simulink model "aves"  (R2012b)
settings: Solver=ode45  StartTime=0.0  StopTime=10.0  RelTol=1e-3
undefined symbols (not defined in the file): ave
settings Model: Creator=Daniel  LastModifiedBy=Daniel

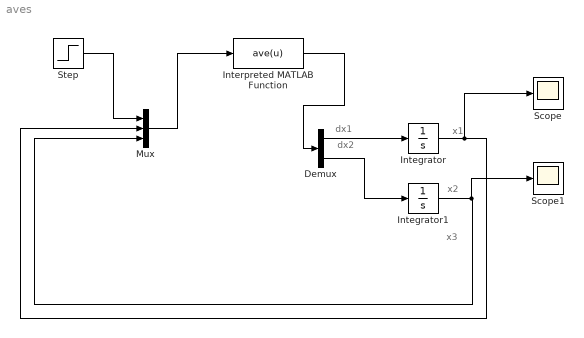
== system aves ==
  note: x3
  note: x2
  note: x1
  note: dx2
  note: dx1
  Demux : Demux  Outputs=2
  Integrator : Integrator
  Integrator1 : Integrator
  Interpreted MATLAB Function : MATLABFcn  MATLABFcn=ave(u)  OutputDimensions=2
  Mux : Mux  Inputs=3
  Scope : Scope
  Scope1 : Scope
  Step : Step  After=6  SampleTime=0
  wires:
  Interpreted MATLAB Function/1 -> Demux/1
  Mux/1 -> Interpreted MATLAB Function/1
  Demux/1 -> Integrator/1
  Demux/2 -> Integrator1/1
  Integrator1/1 -> Scope1/1, Mux/3
  Integrator/1 -> Scope/1, Mux/2
  Step/1 -> Mux/1
